simulink model "trkwhlmdldynf"  (R2021a)
settings: Solver=VariableStepAuto  StartTime=0.0  StopTime=20  FixedStep=0.1  RelTol=1e-3
InitFcn:
  | if ~exist("omegal","var")
  |     omegal = 5;
  |     omegar = 5;
  | end
libraries: autolibshared x1, simulink x1
settings Model: LastModifiedBy=polonium

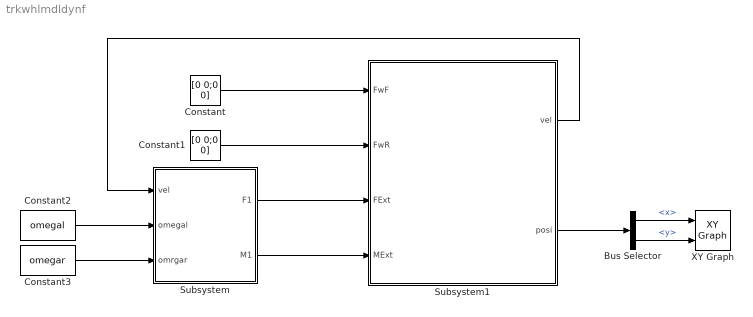
== system trkwhlmdldynf ==
  Bus Selector : BusSelector  OutputSignals=x,y
  Constant : Constant  Value=[0 0;0 0]
  Constant1 : Constant  Value=[0 0;0 0]
  Constant2 : Constant  Value=omegal
  Constant3 : Constant  Value=omegar
  Subsystem : Subsystem  mask{x_mesh=0, y_mesh_l=0, y_mesh_r=0, m=0, trackwidth=0, trackgap=0, mu=0, K=0, r=0, l=0}
      mask prompts: x_mesh "x mesh"; y_mesh_l "left y mesh"; y_mesh_r "right y mesh"; m "vehicle mass"; trackwidth "track width"; trackgap "track latral distance"; mu "soil parameter mu"; K "soil parameter K"; r "track drive wheel radius"; l "track length"
  Subsystem1 : Subsystem
  XY Graph : simulink/Sinks/XY Graph  xmin=-10  xmax=10  ymin=-10  ymax=10  st=-1
  wires:
  Bus Selector/1 -> XY Graph/1  "<x>"
  Bus Selector/2 -> XY Graph/2  "<y>"
  Constant2/1 -> Subsystem/2(omegal)
  Constant3/1 -> Subsystem/3(omrgar)
  Constant/1 -> Subsystem1/1(FwF)
  Constant1/1 -> Subsystem1/2(FwR)
  Subsystem/1(F1) -> Subsystem1/3(FExt)
  Subsystem/2(M1) -> Subsystem1/4(MExt)
  Subsystem1/1(vel) -> Subsystem/1(vel)
  Subsystem1/2(posi) -> Bus Selector/1

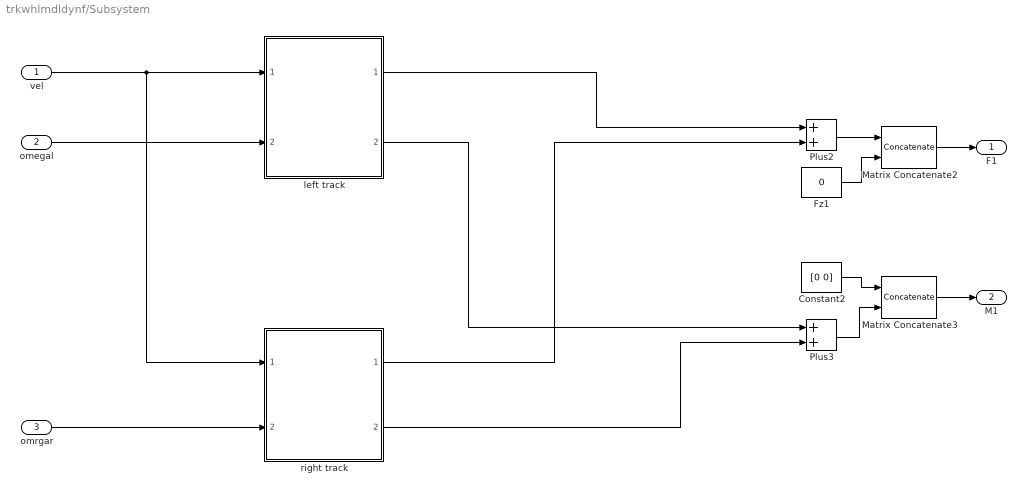
== system trkwhlmdldynf/Subsystem ==
  vel : Inport
  omegal : Inport  Port=2
  omrgar : Inport  Port=3
  Constant2 : Constant  Value=[0 0]  VectorParams1D=off
  Fz1 : Constant  Value=0
  Matrix Concatenate2 : Concatenate  Mode=Multidimensional array  ConcatenateDimension=2
  Matrix Concatenate3 : Concatenate  Mode=Multidimensional array  ConcatenateDimension=2
  Plus2 : Sum
  Plus3 : Sum
  left track : Subsystem  ReferencedSubsystem=singleTrackDynF  leftORright=left track  m=500  trackwidth=0.3  trackgap=0.8  mu=0.5  K=0.2  r=0.3  l=1  xMeshSize=20  yMeshSize=5
  right track : Subsystem  ReferencedSubsystem=singleTrackDynF  leftORright=right track  m=500  trackwidth=0.3  trackgap=0.8  mu=0.5  K=0.2  r=0.3  l=1  xMeshSize=10  yMeshSize=5
  F1 : Outport
  M1 : Outport  Port=2
  wires:
  Matrix Concatenate3/1 -> M1/1
  Plus3/1 -> Matrix Concatenate3/2
  Plus2/1 -> Matrix Concatenate2/1
  left track/2 -> Plus3/1
  Fz1/1 -> Matrix Concatenate2/2
  Constant2/1 -> Matrix Concatenate3/1
  left track/1 -> Plus2/1
  Matrix Concatenate2/1 -> F1/1
  vel/1 -> right track/1, left track/1
  omegal/1 -> left track/2
  omrgar/1 -> right track/2
  right track/1 -> Plus2/2
  right track/2 -> Plus3/2

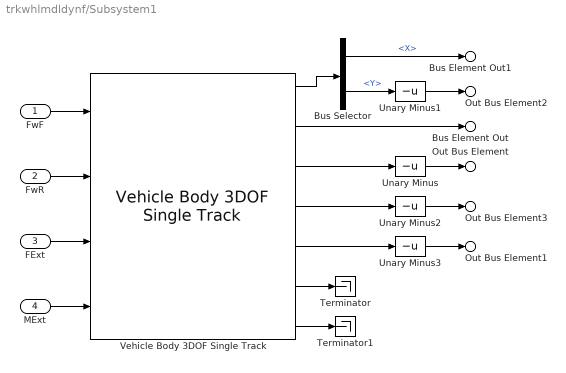
== system trkwhlmdldynf/Subsystem1 ==
  FwF : Inport
  FwR : Inport  Port=2
  FExt : Inport  Port=3
  MExt : Inport  Port=4
  Bus Selector : BusSelector  OutputSignals=InertFrm.Cg.Disp.X,InertFrm.Cg.Disp.Y
  Terminator : Terminator
  Terminator1 : Terminator
  Unary Minus{,1..3} (4 alike) : UnaryMinus
  Vehicle Body 3DOF Single Track : autolibshared/Vehicle Body 3DOF Single Track  trackMode=Dual  inputMode=External forces  frontSteerMode=off  rearSteerMode=off  windMode=off  muMode=off  extFMode=on  extMMode=on  htchFMode=off  htchMMode=off  extXo=off  extpsio=off  extxdoto=off  extro=off  extYo=off  extTamb=off  extydoto=off  aMode=2  NF=2  NR=2  m=500  a=1.4  b=1.6  h=0.35  dh=1  hh=0.2  X_o=0  xdot_o=1.6  CalphaMode=off  sigmaMode=on  d=0  hl=0  w=[1.4,1.4]  Cy_f=12e3  Cy_r=11e3  sigma_f=.1  sigma_r=.1  alpha_f_brk=[-.1 .1]  Cy_f_data=[-9e3 9e3]  alpha_r_brk=[-.1 .1]  Cy_r_data=[-9e3 9e3]  Y_o=0  ydot_o=0  Izz=1000  psi_o=0  r_o=0  Af=2  Cd=.3  Cl=.1  Cpm=.1  beta_w=[0:0.01:0.3]  Cs=[0:0.03:0.9]  Cym=[0:0.01:0.3]  Pabs=101325  Tair=273  g=9.81  mu=1  xdot_tol=.01  Fznom=5000  Fxtire_sat=7e4  Fytire_sat=7e4  longOff=0  latOff=0  vertOff=0  wrapAng=off
      settings: SourceProductBaseCode=PW,DR,MT,UV,VE
  Bus Element Out : Outport  PortName=vel  Element=vx
  Out Bus Element : Outport  PortName=vel  Element=vy
  Out Bus Element1 : Outport  PortName=vel  Element=omegaz
  Bus Element Out1 : Outport  Port=2  PortName=posi  Element=x
  Out Bus Element2 : Outport  Port=2  PortName=posi  Element=y
  Out Bus Element3 : Outport  Port=2  PortName=posi  Element=psi
  wires:
  FwR/1 -> Vehicle Body 3DOF Single Track/2
  Vehicle Body 3DOF Single Track/1 -> Bus Selector/1
  Unary Minus2/1 -> Out Bus Element3/1
  Unary Minus1/1 -> Out Bus Element2/1
  Bus Selector/2 -> Unary Minus1/1  "<Y>"
  MExt/1 -> Vehicle Body 3DOF Single Track/4
  Bus Selector/1 -> Bus Element Out1/1  "<X>"
  FExt/1 -> Vehicle Body 3DOF Single Track/3
  Unary Minus3/1 -> Out Bus Element1/1
  Vehicle Body 3DOF Single Track/3 -> Unary Minus/1
  Unary Minus/1 -> Out Bus Element/1
  FwF/1 -> Vehicle Body 3DOF Single Track/1
  Vehicle Body 3DOF Single Track/2 -> Bus Element Out/1
  Vehicle Body 3DOF Single Track/7 -> Terminator1/1
  Vehicle Body 3DOF Single Track/4 -> Unary Minus2/1
  Vehicle Body 3DOF Single Track/5 -> Unary Minus3/1
  Vehicle Body 3DOF Single Track/6 -> Terminator/1
